simulink model "pmsm_model_Lab4_sensorless_st_R2020a"  (R2023a)
settings: Solver=ode4  StartTime=0.0  StopTime=Tf  FixedStep=Tsim  MaxStep=Tsim  MinStep=Tsim/100  RelTol=1e-3
values from neighbouring files (symbols this model uses):
  b = 0    [pmsm_param_Lab4_2024_st.m]
  C32 = [ 1       0 ... (first row only)    [pmsm_param_Lab4_2024_st.m]
  C32inv = 2/3*[1    -1/2        -1/2 ... (first row only)    [pmsm_param_Lab4_2024_st.m]
  C33 = C32*C32inv    [pmsm_param_Lab4_2024_st.m]
  Cb = 500e-6    (= 0.0005)    [pmsm_param_Lab4_2024_st.m]
  dTm0 = Tmrated/2    (= 120)    [pmsm_param_Lab4_2024_st.m]
  Dyno = 0    [pmsm_param_Lab4_2024_st.m]
  f = 15e-3    (= 0.015)    [pmsm_param_Lab4_2024_st.m]
  frslvr = 1/Ts    (= 10000)    [pmsm_param_Lab4_2024_st.m]
  Id0 = interp1(Tref,Idopt,Tm0)    [pmsm_param_Lab4_2024_st.m]
  Idc0 = Pe0/VDC    [pmsm_param_Lab4_2024_st.m]
  Idopt = zeros(1,NT)    [pmsm_param_Lab4_2024_st.m]
  Iq0 = interp1(Tref,Iqopt,Tm0)    [pmsm_param_Lab4_2024_st.m]
  Iqopt = zeros(1,NT)    [pmsm_param_Lab4_2024_st.m]
  J = 100e-3    (= 0.1)    [pmsm_param_Lab4_2024_st.m]
  Kid = Kpd/tid    (= 180)    [pmsm_param_Lab4_2024_st.m]
  Kiq = Kpq/tiq    (= 180)    [pmsm_param_Lab4_2024_st.m]
  kL = 0.750    (= 0.75)    [pmsm_param_Lab4_2024_st.m]
  Kpd = 3*Ld0/tr    (= 3)    [pmsm_param_Lab4_2024_st.m]
  Kpll = 760    [pmsm_param_Lab4_2024_st.m]
  Kpq = 3*Lq0/tr    (= 6)    [pmsm_param_Lab4_2024_st.m]
  ksi = 0    [pmsm_param_Lab4_2024_st.m]
  Lb = 20e-6    (= 2e-05)    [pmsm_param_Lab4_2024_st.m]
  Ld0 = 1.0*Ld    (= 0.001)    [pmsm_param_Lab4_2024_st.m]
  Lq0 = 1.0*Lq    (= 0.002)    [pmsm_param_Lab4_2024_st.m]
  Pe0 = 3/2*(Vd0*Id0+Vq0*Iq0)    [pmsm_param_Lab4_2024_st.m]
  Pp = 4    [pmsm_param_Lab4_2024_st.m]
  ppll = cell2mat(ppll)    [pmsm_param_Lab4_2024_st.m]
  Psid0 = interpn(Idv,Iqv,Psidd,Id0,Iq0)    [pmsm_param_Lab4_2024_st.m]
  Psif0 = 1.0*Psif    (= 0.167)    [pmsm_param_Lab4_2024_st.m]
  Psiq0 = interpn(Idv,Iqv,Psiqq,Id0,Iq0)    [pmsm_param_Lab4_2024_st.m]
  Qbat = 72*3600    (= 259200)    [pmsm_param_Lab4_2024_st.m]
  RateTm = 10000    [pmsm_param_Lab4_2024_st.m]
  rb = 80e-3    (= 0.08)    [pmsm_param_Lab4_2024_st.m]
  Rs = 60e-3    (= 0.06)    [pmsm_param_Lab4_2024_st.m]
  Rs0 = 1.0*Rs    (= 0.06)    [pmsm_param_Lab4_2024_st.m]
  SOC0 = 0.50    (= 0.5)    [pmsm_param_Lab4_2024_st.m]
  Thetae0 = 0    [pmsm_param_Lab4_2024_st.m]
  Tm0 = (kL+f)*Wm0    (= 0)    [pmsm_param_Lab4_2024_st.m]
  Tp = 100e-6    (= 0.0001)    [pmsm_param_Lab4_2024_st.m]
  Tref = -Tmax:Tmax/100:Tmax    [pmsm_param_Lab4_2024_st.m]
  Ts = Tp    (= 0.0001)    [pmsm_param_Lab4_2024_st.m]
  Tsim = min([Tp Ts])/100    [pmsm_param_Lab4_2024_st.m]
  TSS = Tstep+0.050    (= 0.1)    [pmsm_param_Lab4_2024_st.m]
  Tstep = 0.050    (= 0.05)    [pmsm_param_Lab4_2024_st.m]
  Ud0 = Rs*Id0    (= 0)    [pmsm_param_Lab4_2024_st.m]
  Uq0 = Rs*Iq0    [pmsm_param_Lab4_2024_st.m]
  Vd0 = Ud0-Pp*Psiq0*Wm0    [pmsm_param_Lab4_2024_st.m]
  VDC = 800    [pmsm_param_Lab4_2024_st.m]
  VDC0 = 0.8*VDC    (= 640)    [pmsm_param_Lab4_2024_st.m]
  Vp = VDC/2    (= 400)    [pmsm_param_Lab4_2024_st.m]
  Vq0 = Uq0+Pp*Psid0*Wm0    [pmsm_param_Lab4_2024_st.m]
  we0 = Pp*Wm0    (= 0)    [pmsm_param_Lab4_2024_st.m]
  Wm0 = 3000*pi/30*0    (= 0)    [pmsm_param_Lab4_2024_st.m]
  zpll = cell2mat(zpll)    [pmsm_param_Lab4_2024_st.m]
undefined symbols (not defined in the file or in its folder): DiscIntNeverNeededParam, Idd, Idrop, Iqq, Isw, kpll, Psidv, Psiqv, SwLoss, Vdrop
libraries: simulink x10
(part 2 of 2)

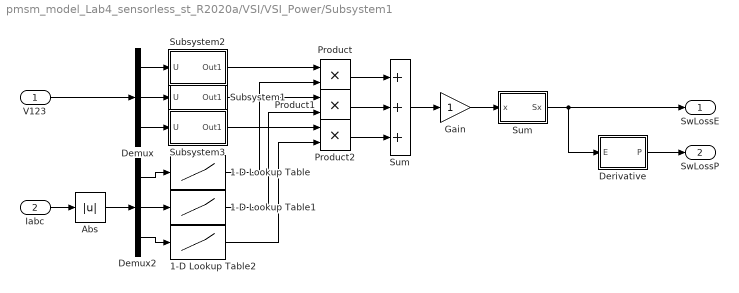
== system pmsm_model_Lab4_sensorless_st_R2020a/VSI/VSI_Power/Subsystem1 ==
  V123 : Inport
  Iabc : Inport  Port=2
  1-D Lookup Table : Lookup_n-D  NumberOfTableDimensions=1  BreakpointsForDimension1=Isw  Table=SwLoss  InternalRulePriority=Speed  RndMeth=Simplest
  1-D Lookup Table1 : Lookup_n-D  NumberOfTableDimensions=1  BreakpointsForDimension1=Isw  Table=SwLoss  InternalRulePriority=Speed  RndMeth=Simplest
  1-D Lookup Table2 : Lookup_n-D  NumberOfTableDimensions=1  BreakpointsForDimension1=Isw  Table=SwLoss  InternalRulePriority=Speed  RndMeth=Simplest
  Abs : Abs  SaturateOnIntegerOverflow=off
  Demux : Demux  Outputs=3
  Demux2 : Demux  Outputs=3
  Derivative : Subsystem
  Gain : Gain
  Product : Product
  Product1 : Product
  Product2 : Product
  Subsystem1 : Subsystem
  Subsystem2 : Subsystem
  Subsystem3 : Subsystem
  Sum : Sum  Inputs=+++
  "Sum " : Subsystem
  SwLossE : Outport
  SwLossP : Outport  Port=2
  wires:
  V123/1 -> Demux/1
  Abs/1 -> Demux2/1
  Demux2/3 -> 1-D Lookup Table2/1
  Demux2/2 -> 1-D Lookup Table1/1
  Demux2/1 -> 1-D Lookup Table/1
  Product2/1 -> Sum/3
  Product1/1 -> Sum/2
  Product/1 -> Sum/1
  Subsystem1/1(Out1) -> Product1/1
  Subsystem3/1(Out1) -> Product2/1
  Iabc/1 -> Abs/1
  Sum/1 -> Gain/1
  Subsystem2/1(Out1) -> Product/1
  Demux/3 -> Subsystem3/1(U)
  Demux/2 -> Subsystem1/1(U)
  Demux/1 -> Subsystem2/1(U)
  1-D Lookup Table/1 -> Product/2
  1-D Lookup Table1/1 -> Product1/2
  1-D Lookup Table2/1 -> Product2/2
  Derivative/1(P) -> SwLossP/1
  "Sum "/1(Sx) -> Derivative/1(E), SwLossE/1
  Gain/1 -> "Sum "/1(x)

== system pmsm_model_Lab4_sensorless_st_R2020a/VSI/VSI_Power/Subsystem1/Derivative ==
  E : Inport
  Divide1 : Product  Inputs=/*
  Saturation : Saturate  UpperLimit=inf  LowerLimit=1e-9
  Sum2 : Sum  Inputs=|+-
  Sum5 : Sum  Inputs=+-|
  Unit Delay1 : UnitDelay  SampleTime=-1  HasFrameUpgradeWarning=on
  Unit Delay2 : UnitDelay  SampleTime=-1  HasFrameUpgradeWarning=on
  P : Outport
  wires:
  Unit Delay2/1 -> Sum5/2
  Saturation/1 -> Divide1/1
  [Clk] -> Sum5/1, Unit Delay2/1
  E/1 -> Unit Delay1/1, Sum2/1
  Unit Delay1/1 -> Sum2/2
  Sum5/1 -> Saturation/1
  Sum2/1 -> Divide1/2
  Divide1/1 -> P/1

== system pmsm_model_Lab4_sensorless_st_R2020a/VSI/VSI_Power/Subsystem1/Subsystem1 ==
  U : Inport
  Gain : Gain
  Gain1 : Gain
  Subsystem : Subsystem
  Subsystem1 : Subsystem
  Sum3 : Sum  Inputs=|++  SaturateOnIntegerOverflow=on
  Out1 : Outport
  wires:
  U/1 -> Subsystem/1(U), Subsystem1/1(U)
  Subsystem1/1(Out1) -> Gain1/1
  Subsystem/1(Out1) -> Gain/1
  Gain/1 -> Sum3/2
  Sum3/1 -> Out1/1
  Gain1/1 -> Sum3/1

== system pmsm_model_Lab4_sensorless_st_R2020a/VSI/VSI_Power/Subsystem1/Subsystem2 ==
  U : Inport
  Gain : Gain
  Gain1 : Gain
  Subsystem : Subsystem
  Subsystem1 : Subsystem
  Sum3 : Sum  Inputs=|++  SaturateOnIntegerOverflow=on
  Out1 : Outport
  wires:
  Gain1/1 -> Sum3/1
  Sum3/1 -> Out1/1
  Gain/1 -> Sum3/2
  Subsystem/1(Out1) -> Gain/1
  Subsystem1/1(Out1) -> Gain1/1
  U/1 -> Subsystem1/1(U), Subsystem/1(U)

== system pmsm_model_Lab4_sensorless_st_R2020a/VSI/VSI_Power/Subsystem1/Subsystem3 ==
  U : Inport
  Gain : Gain
  Gain1 : Gain
  Subsystem : Subsystem
  Subsystem1 : Subsystem
  Sum3 : Sum  Inputs=|++  SaturateOnIntegerOverflow=on
  Out1 : Outport
  wires:
  Gain1/1 -> Sum3/1
  Sum3/1 -> Out1/1
  Gain/1 -> Sum3/2
  Subsystem/1(Out1) -> Gain/1
  Subsystem1/1(Out1) -> Gain1/1
  U/1 -> Subsystem1/1(U), Subsystem/1(U)

== system pmsm_model_Lab4_sensorless_st_R2020a/VSI/VSI_Power/Subsystem1/Sum  ==
  x : Inport
  Memory : Memory
  Sum1 : Sum  Inputs=|++
  Sx : Outport
  wires:
  Memory/1 -> Sum1/2
  x/1 -> Sum1/1
  Sum1/1 -> Memory/1, Sx/1

== system pmsm_model_Lab4_sensorless_st_R2020a/VSI/VSI_Power/Subsystem1/Subsystem1/Subsystem ==
  U : Inport
  Compare To Constant : simulink/Logic and Bit Operations/Compare To Constant  relop=<  const=-VDC0  OutDataTypeStr=uint8
  Memory : Memory
  Sum : Sum  Inputs=+-|
  Out1 : Outport
  wires:
  Compare To Constant/1 -> Out1/1
  U/1 -> Sum/1, Memory/1
  Sum/1 -> Compare To Constant/1
  Memory/1 -> Sum/2

== system pmsm_model_Lab4_sensorless_st_R2020a/VSI/VSI_Power/Subsystem1/Subsystem1/Subsystem1 ==
  U : Inport
  Compare To Constant : simulink/Logic and Bit Operations/Compare To Constant  relop=>  const=VDC0  OutDataTypeStr=uint8
  Memory : Memory
  Sum : Sum  Inputs=+-|
  Out1 : Outport
  wires:
  Compare To Constant/1 -> Out1/1
  Memory/1 -> Sum/2
  Sum/1 -> Compare To Constant/1
  U/1 -> Sum/1, Memory/1

== system pmsm_model_Lab4_sensorless_st_R2020a/VSI/VSI_Power/Subsystem1/Subsystem2/Subsystem ==
  U : Inport
  Compare To Constant : simulink/Logic and Bit Operations/Compare To Constant  relop=<  const=-VDC0  OutDataTypeStr=uint8
  Memory : Memory
  Sum : Sum  Inputs=+-|
  Out1 : Outport
  wires:
  Memory/1 -> Sum/2
  Sum/1 -> Compare To Constant/1
  U/1 -> Memory/1, Sum/1
  Compare To Constant/1 -> Out1/1

== system pmsm_model_Lab4_sensorless_st_R2020a/VSI/VSI_Power/Subsystem1/Subsystem2/Subsystem1 ==
  U : Inport
  Compare To Constant : simulink/Logic and Bit Operations/Compare To Constant  relop=>  const=VDC0  OutDataTypeStr=uint8
  Memory : Memory
  Sum : Sum  Inputs=+-|
  Out1 : Outport
  wires:
  U/1 -> Memory/1, Sum/1
  Sum/1 -> Compare To Constant/1
  Memory/1 -> Sum/2
  Compare To Constant/1 -> Out1/1

== system pmsm_model_Lab4_sensorless_st_R2020a/VSI/VSI_Power/Subsystem1/Subsystem3/Subsystem ==
  U : Inport
  Compare To Constant : simulink/Logic and Bit Operations/Compare To Constant  relop=<  const=-VDC0  OutDataTypeStr=uint8
  Memory : Memory
  Sum : Sum  Inputs=+-|
  Out1 : Outport
  wires:
  Memory/1 -> Sum/2
  Sum/1 -> Compare To Constant/1
  U/1 -> Memory/1, Sum/1
  Compare To Constant/1 -> Out1/1

== system pmsm_model_Lab4_sensorless_st_R2020a/VSI/VSI_Power/Subsystem1/Subsystem3/Subsystem1 ==
  U : Inport
  Compare To Constant : simulink/Logic and Bit Operations/Compare To Constant  relop=>  const=VDC0  OutDataTypeStr=uint8
  Memory : Memory
  Sum : Sum  Inputs=+-|
  Out1 : Outport
  wires:
  U/1 -> Memory/1, Sum/1
  Sum/1 -> Compare To Constant/1
  Memory/1 -> Sum/2
  Compare To Constant/1 -> Out1/1

== matlab function pmsm_model_Lab4_sensorless_st_R2020a/Control/DiscreteR//D/PLL/MATLAB Function ==
  data: u input; y output
function y = fcn(u)

y=atan2(u(1),u(2));  % 2pi-arctangent PLL

== matlab function pmsm_model_Lab4_sensorless_st_R2020a/Control/Ctrl ==
  data: idref input; idm input; iqref input; iqm input; we input; Pp parameter; Psif0 parameter; Ld0 parameter; Lq0 parameter; Rs0 parameter; Ts parameter; vd output; vq output; Kpd parameter; Kpq parameter; Kid parameter; Kiq parameter; Id0 parameter; Iq0 parameter; Ud0 parameter; Uq0 parameter; Tm0 parameter; Vd0 parameter; Vq0 parameter
function [vd, vq]  = Ctrl(idref, idm, iqref, iqm, we, Pp, Psif0, Ld0, Lq0, Rs0, Ts, Kpd, Kpq, Kid, Kiq, Id0, Iq0, Ud0, Uq0, Tm0, Vd0, Vq0)

persistent interrd interrq 

if isempty(interrd), interrd = Ud0; end
if isempty(interrq), interrq = Uq0; end

errd=idref-idm;
errq=iqref-iqm;
interrd=interrd+Kid*errd*Ts;
interrq=interrq+Kiq*errq*Ts;
vd=Kpd*errd+interrd-Lq0*iqm*we;
vq=Kpq*errq+interrq+(Psif0+Ld0*idm)*we;

end

== matlab function pmsm_model_Lab4_sensorless_st_R2020a/Control/sensorless/MATLAB Function ==
  data: v input size=2; i input size=2; w input size=1; e output size=2; Rs0 parameter; Ld0 parameter; Lq0 parameter; Psif0 parameter; Thetae0 parameter; we0 parameter
function e = fcn(v, i, w, Rs0, Ld0, Lq0, Psif0, Thetae0, we0)

persistent edf egf 

if isempty(edf), edf=0; end
if isempty(egf), egf=0; end

ed=0;
eg=0;

adf=0.95;
agf=0.98;
edf=adf*edf+(1-adf)*ed;
egf=agf*egf+(1-agf)*eg;

e=[edf; egf];

== matlab function pmsm_model_Lab4_sensorless_st_R2020a/Control/sensorless/MATLAB Function1 ==
  data: e input; ws output; b parameter; Psif0 parameter; ksi parameter
function ws = fcn(e, b, Psif0, ksi)

ed=e(1);
eg=e(2);

Kp=b/Psif0*(1-ksi*sign(ed));%*sign(eg);
es=sqrt(ed^2+eg^2);
X=ed/(es+eg+1e-3);

% ws=eg/Psif0-Kp*ed; % conventional sensorless
% ws=eg/Psif0-2*Kp*X*es; % half-tangent sensorless
% ws=eg/Psif0-2*Kp*atan(X)*es; % arctangent sensorless
ws=eg/Psif0-Kp*atan2(ed,eg)*es; % 2pi-arctangent sensorless

== matlab function pmsm_model_Lab4_sensorless_st_R2020a/PMSM/dq-PMSM ==
  data: vd input; dPsid output; vq input; id input; iq input; Psid input; Psiq input; Omega input; TL input; dPsiq output; dOmega output; dTheta output; Rs input; Pp parameter; f parameter; J parameter; Tm output
function [dPsid, dPsiq, dOmega, dTheta, Tm] = PMSM(vd, vq, id, iq, Psid, Psiq, Omega, TL, Rs, Pp, f, J)

w=Pp*Omega;
Tm=(3/2)*Pp*(Psid*iq-Psiq*id);   % Clarke
% Tm=p*(Psid*iq-Psiq*id);       % Concordia

dPsid=vd-Rs*id+w*Psiq;
dPsiq=vq-Rs*iq-w*Psid;
dOmega=(Tm-f*Omega-TL)/J;
dTheta=w;

== matlab function pmsm_model_Lab4_sensorless_st_R2020a/Control/DiscreteR//D/MATLAB Function ==
  settings: updateMethod=DISCRETE
  data: c input; s input; F output; w input
function F = fcn(c, s, w)

F=0;
